simulink model "controller_tuner"  (R2016a)
settings: Solver=FixedStepDiscrete  StartTime=0.0  StopTime=inf  FixedStep=0.001  RelTol=1e-3
undefined symbols (not defined in the file or in its folder): Left_Leg
libraries: xpcethercatlib x14, slrtlib x5, simulink x2
settings Model: xpc_rtwmakecfg_data=_xpcethercatlib_  SimulationMode=external  Creator=Projectmarch  LastModifiedBy=Projectmarch
settings SolverCC: EnableConcurrentExecution=on
settings DataIOCC: SaveFormat=StructureWithTime
settings OptimizationCC: BlockReduction=off  OptimizeBlockIOStorage=off  BufferReuse=off  GlobalBufferReuse=off  ExpressionFolding=off  LocalBlockOutputs=off
settings HardwareCC: ProdBitPerPointer=32  ProdLargestAtomicFloat=None  ProdWordSize=32  ProdLongLongMode=on  ProdHWDeviceType=Generic->32-bit x86 compatible
settings RTWCC: SystemTargetFile=slrt.tlc  TemplateMakefile=slrt_default_tmf  Description=Simulink Real-Time  RTWCompilerOptimization=on

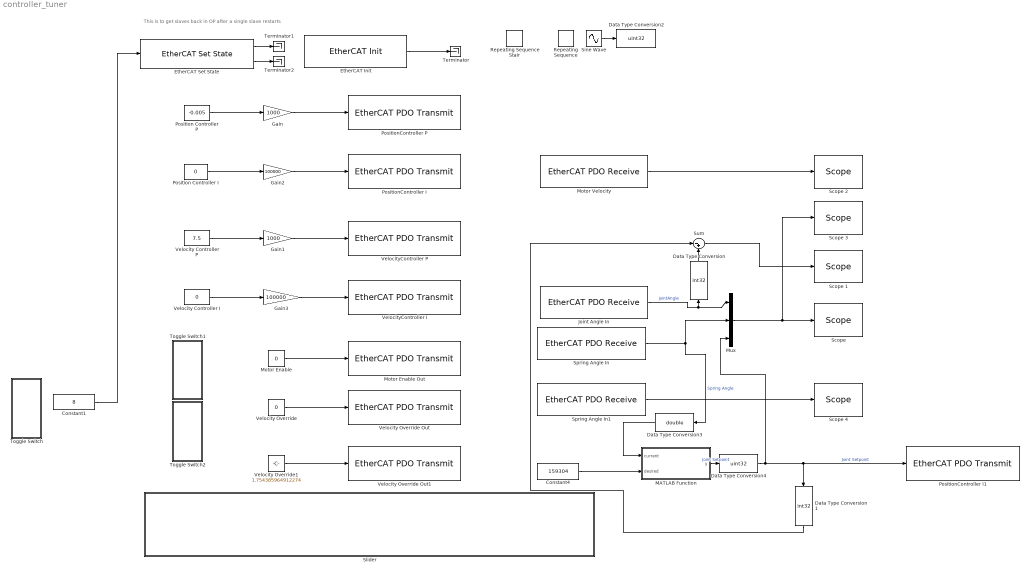
== system controller_tuner ==
  note: This is to get slaves back in OP after a single slave restarts
  Constant1 : Constant  Value=8  OutDataTypeStr=Inherit: Inherit via back propagation
  Constant4 : Constant  Value=159304  OutDataTypeStr=Inherit: Inherit via back propagation
  Data Type Conversion : DataTypeConversion  OutDataTypeStr=int32
  Data Type Conversion1 : DataTypeConversion  OutDataTypeStr=int32
  Data Type Conversion2 : DataTypeConversion  OutDataTypeStr=uint32
  Data Type Conversion3 : DataTypeConversion  OutDataTypeStr=double
  Data Type Conversion4 : DataTypeConversion  OutDataTypeStr=uint32
  "EtherCAT Init " : xpcethercatlib/EtherCAT Init   Priority=0  config_file=D:\Software\MATLAB\simulink-models\EtherCAT Config files\full_setup_v1.0.xml  device_id=0  pci_bus=2  pci_slot=0  dctuning=2  enaDebug=off  enaDC=on  errLink=off  masterDbg=off  stateChgDbg=off  baseClock=off  masterCfg=off  logFile='c:\dbglog.txt'  sample_time=0.001000
  "EtherCAT Set State " : xpcethercatlib/EtherCAT Set State   device_id=0  timeout=0  sample_time=0
  Gain : Gain  Gain=1000  OutDataTypeStr=Inherit: Inherit via back propagation
  Gain1 : Gain  Gain=1000  OutDataTypeStr=Inherit: Inherit via back propagation
  Gain2 : Gain  Gain=100000  OutDataTypeStr=Inherit: Inherit via back propagation
  Gain3 : Gain  Gain=100000  OutDataTypeStr=Inherit: Inherit via back propagation
  Joint Angle In : xpcethercatlib/EtherCAT PDO Receive  Priority=2  sig_name=Left_Leg.Inputs.H_jointAngle  sig_offset=1144  sig_type=uint32  type_size=32  sig_dim=1  device_id=0  sample_time=0.001000
  MATLAB Function : MATLAB Function  TreatAsAtomicUnit=on
  Motor Enable : Constant  Value=0  OutDataTypeStr=Inherit: Inherit via back propagation
  Motor Enable Out : xpcethercatlib/EtherCAT PDO Transmit   Priority=3  sig_name=Left_Leg.Outputs.H_motorEnable  sig_offset=1192  sig_type=uint8  type_size=8  sig_dim=1  device_id=0  sample_time=0.001000
  Motor Velocity : xpcethercatlib/EtherCAT PDO Receive  Priority=2  sig_name=Left_Leg.Inputs.H_motorVelocity  sig_offset=1224  sig_type=int16  type_size=16  sig_dim=1  device_id=0  sample_time=0.001000
  Mux : Mux  Inputs=3
  Position Controller I : Constant  Value=0
  Position Controller P : Constant  Value=-0.005
  PositionController I : xpcethercatlib/EtherCAT PDO Transmit   Priority=3  sig_name=Left_Leg.Outputs.H_data[1]  sig_offset=1304  sig_type=int32  type_size=32  sig_dim=1  device_id=0  sample_time=0.001000
  PositionController I1 : xpcethercatlib/EtherCAT PDO Transmit   Priority=3  sig_name=Left_Leg.Outputs.H_jointSetPoint  sig_offset=1160  sig_type=uint32  type_size=32  sig_dim=1  device_id=0  sample_time=0.001000
  PositionController P : xpcethercatlib/EtherCAT PDO Transmit   Priority=3  sig_name=Left_Leg.Outputs.H_data[0]  sig_offset=1272  sig_type=int32  type_size=32  sig_dim=1  device_id=0  sample_time=0.001000
  Repeating Sequence : simulink/Sources/Repeating Sequence  rep_seq_t=[0 2]  rep_seq_y=[0 2]
  Repeating Sequence Stair : simulink/Sources/Repeating Sequence Stair  OutValues=[3 1 4 2 1].'  tsamp=-1  OutMin=[]  OutMax=[]  OutDataTypeStr=double  OutputDataTypeScalingMode=double  OutDataType=fixdt(0,8)  ConRadixGroup=Best Precision: Vector-wise  OutScaling=2^-12
  "Scope " : slrtlib/Displays and Logging/Scope   scopeno=1  scopetype=Target  autostart=on  viewmode=Graphical sliding  formatstr='%15.6f'  grid=on  ylimits=[0,0]  nosamples=10000  noprepostsamples=0  interleave=1  triggermode=FreeRun  triggersignal=1  trigsignalfromport=off  triggerlevel=0.0  triggerslope=Either  triggerscope=1  triggersample=0  filename=data.dat  mode=Lazy  writesize=512  autorestart=off  dynamicfilemode=off  maxwritefilesize=512*1024^2
  Scope 1 : slrtlib/Displays and Logging/Scope   scopeno=2  scopetype=Target  autostart=on  viewmode=Graphical sliding  formatstr='%15.6f'  grid=on  ylimits=[0,0]  nosamples=10000  noprepostsamples=0  interleave=1  triggermode=FreeRun  triggersignal=1  trigsignalfromport=off  triggerlevel=0.0  triggerslope=Either  triggerscope=1  triggersample=0  filename=data.dat  mode=Lazy  writesize=512  autorestart=off  dynamicfilemode=off  maxwritefilesize=512*1024^2
  Scope 2 : slrtlib/Displays and Logging/Scope   scopeno=3  scopetype=Target  autostart=on  viewmode=Graphical sliding  formatstr='%15.6f'  grid=on  ylimits=[0,0]  nosamples=10000  noprepostsamples=0  interleave=1  triggermode=FreeRun  triggersignal=1  trigsignalfromport=off  triggerlevel=0.0  triggerslope=Either  triggerscope=1  triggersample=0  filename=data.dat  mode=Lazy  writesize=512  autorestart=off  dynamicfilemode=off  maxwritefilesize=512*1024^2
  Scope 3 : slrtlib/Displays and Logging/Scope   scopeno=4  scopetype=Target  autostart=on  viewmode=Numerical  formatstr='%15.6f'  grid=on  ylimits=[0,0]  nosamples=250  noprepostsamples=0  interleave=1  triggermode=FreeRun  triggersignal=1  trigsignalfromport=off  triggerlevel=0.0  triggerslope=Either  triggerscope=1  triggersample=0  filename=data.dat  mode=Lazy  writesize=512  autorestart=off  dynamicfilemode=off  maxwritefilesize=512*1024^2
  Scope 4 : slrtlib/Displays and Logging/Scope   scopeno=5  scopetype=Target  autostart=on  viewmode=Graphical sliding  formatstr='%15.6f'  grid=on  ylimits=[0,0]  nosamples=10000  noprepostsamples=0  interleave=1  triggermode=FreeRun  triggersignal=1  trigsignalfromport=off  triggerlevel=0.0  triggerslope=Either  triggerscope=1  triggersample=0  filename=data.dat  mode=Lazy  writesize=512  autorestart=off  dynamicfilemode=off  maxwritefilesize=512*1024^2
  Sine Wave : Sin  Amplitude=20000  Bias=370000  Frequency=2  SampleTime=0.001
  Slider : Subsystem  DialogController=hmiCreateDDGDialog  IsWebBlock=on  mask(MWDashboardBlock){webBlockId=69257127-0cdf-46c0-968c-0481a6079d56, webBlockType=slider, ShowInLibBrowser=on, ShowInitialText=on, HMISrcModelName=controller_tuner}
      mask prompts: webBlockId "WebBlock Id"; webBlockType "WebBlock Type"; HMISrcModelName "Source Model"
      mask Help: helpview([docroot '/mapfiles/simulink.map'], 'hmi_slider')
      mask Display:
      | if strcmp(get_param(bdroot(gcb),'BlockDiagramType'), 'library')
      |     image([(matlabroot) '/toolbox/simulink/hmi/icons/Slider.png']);
      | end
  Spring Angle In : xpcethercatlib/EtherCAT PDO Receive  Priority=2  sig_name=Left_Leg.Inputs.H_springAngle  sig_offset=1176  sig_type=uint32  type_size=32  sig_dim=1  device_id=0  sample_time=0.001000
  Spring Angle In1 : xpcethercatlib/EtherCAT PDO Receive  Priority=2  sig_name=Left_Leg.Inputs.K_footForceFront[0]  sig_offset=1464  sig_type=int32  type_size=32  sig_dim=1  device_id=0  sample_time=0.001000
  Sum : Sum  Inputs=|-+
  Terminator : Terminator
  Terminator1 : Terminator
  Terminator2 : Terminator
  Toggle Switch : Subsystem  DialogController=hmiCreateDDGDialog  IsWebBlock=on  mask(MWDashboardBlock){webBlockId=7114826d-f1c9-4545-bae4-963e2c516657, webBlockType=toggleswitch, ShowInLibBrowser=on, ShowInitialText=on, HMISrcModelName=controller_tuner}
      mask prompts: webBlockId "WebBlock Id"; webBlockType "WebBlock Type"; HMISrcModelName "Source Model"
      mask Help: helpview([docroot '/mapfiles/simulink.map'], 'hmi_toggle_switch')
      mask Display:
      | if strcmp(get_param(bdroot(gcb),'BlockDiagramType'), 'library')
      |     image([(matlabroot) '/toolbox/simulink/hmi/icons/ToggleSwitch.png']);
      | end
  Toggle Switch1 : Subsystem  DialogController=hmiCreateDDGDialog  IsWebBlock=on  mask(MWDashboardBlock){webBlockId=dae9756d-5b12-44cc-89b0-22c61f9c3f4a, webBlockType=toggleswitch, ShowInLibBrowser=on, ShowInitialText=on, HMISrcModelName=controller_tuner}
      mask prompts: webBlockId "WebBlock Id"; webBlockType "WebBlock Type"; HMISrcModelName "Source Model"
      mask Help: helpview([docroot '/mapfiles/simulink.map'], 'hmi_toggle_switch')
      mask Display:
      | if strcmp(get_param(bdroot(gcb),'BlockDiagramType'), 'library')
      |     image([(matlabroot) '/toolbox/simulink/hmi/icons/ToggleSwitch.png']);
      | end
  Toggle Switch2 : Subsystem  DialogController=hmiCreateDDGDialog  IsWebBlock=on  mask(MWDashboardBlock){webBlockId=6206497e-7561-4c19-9056-57079e110fb5, webBlockType=toggleswitch, ShowInLibBrowser=on, ShowInitialText=on, HMISrcModelName=controller_tuner}
      mask prompts: webBlockId "WebBlock Id"; webBlockType "WebBlock Type"; HMISrcModelName "Source Model"
      mask Help: helpview([docroot '/mapfiles/simulink.map'], 'hmi_toggle_switch')
      mask Display:
      | if strcmp(get_param(bdroot(gcb),'BlockDiagramType'), 'library')
      |     image([(matlabroot) '/toolbox/simulink/hmi/icons/ToggleSwitch.png']);
      | end
  Velocity Controller I : Constant  Value=0
  Velocity Controller P : Constant  Value=7.5
  Velocity Override : Constant  Value=0  OutDataTypeStr=Inherit: Inherit via back propagation
  Velocity Override Out : xpcethercatlib/EtherCAT PDO Transmit   Priority=3  sig_name=Left_Leg.Outputs.H_data[4]  sig_offset=1400  sig_type=int32  type_size=32  sig_dim=1  device_id=0  sample_time=0.001000
  Velocity Override Out1 : xpcethercatlib/EtherCAT PDO Transmit   Priority=3  sig_name=Left_Leg.Outputs.H_velocitySetPoint  sig_offset=1144  sig_type=int16  type_size=16  sig_dim=1  device_id=0  sample_time=0.001000
  Velocity Override1 : Constant  Value=1.754385964912274  OutDataTypeStr=Inherit: Inherit via back propagation
  VelocityController I : xpcethercatlib/EtherCAT PDO Transmit   Priority=3  sig_name=Left_Leg.Outputs.K_data[3]  sig_offset=1656  sig_type=int32  type_size=32  sig_dim=1  device_id=0  sample_time=0.001000
  VelocityController P : xpcethercatlib/EtherCAT PDO Transmit   Priority=3  sig_name=Left_Leg.Outputs.H_data[2]  sig_offset=1336  sig_type=int32  type_size=32  sig_dim=1  device_id=0  sample_time=0.001000
  wires:
  Position Controller P/1 -> Gain/1
  Gain/1 -> PositionController P/1
  Velocity Controller P/1 -> Gain1/1
  Gain1/1 -> VelocityController P/1
  Position Controller I/1 -> Gain2/1
  Velocity Controller I/1 -> Gain3/1
  Gain3/1 -> VelocityController I/1
  Gain2/1 -> PositionController I/1
  Velocity Override/1 -> Velocity Override Out/1
  Motor Enable/1 -> Motor Enable Out/1
  "EtherCAT Init "/1 -> Terminator/1
  Joint Angle In/1 -> Data Type Conversion/1, Mux/1  "jointAngle"
  Spring Angle In/1 -> Mux/2, Data Type Conversion3/1  "Spring Angle"
  Mux/1 -> Scope 3/1, "Scope "/1
  Motor Velocity/1 -> Scope 2/1
  Spring Angle In1/1 -> Scope 4/1
  Sum/1 -> Scope 1/1
  Data Type Conversion1/1 -> Sum/1
  Data Type Conversion/1 -> Sum/2
  Constant4/1 -> MATLAB Function/2(desired)
  Sine Wave/1 -> Data Type Conversion2/1
  "EtherCAT Set State "/1 -> Terminator1/1
  "EtherCAT Set State "/2 -> Terminator2/1
  Constant1/1 -> "EtherCAT Set State "/1
  Velocity Override1/1 -> Velocity Override Out1/1
  MATLAB Function/1(y) -> Data Type Conversion4/1  "Joint Setpoint"
  Data Type Conversion3/1 -> MATLAB Function/1(current)
  Data Type Conversion4/1 -> Mux/3, PositionController I1/1, Data Type Conversion1/1  "Joint Setpoint"

== system controller_tuner/Slider ==

== system controller_tuner/Toggle Switch ==

== system controller_tuner/Toggle Switch1 ==

== system controller_tuner/Toggle Switch2 ==

== matlab function controller_tuner/MATLAB Function ==
  data: current input; y output; desired input
function y = fcn(current,desired)
%#codegen

persistent i desiredPersistent trajectory startup;

f = 700;

if(isempty(trajectory))
   trajectory = [0 0]; 
end

% Send out the current value until desired is changed
if(isempty(startup))
    i = 1;
    startup = 1;
    desiredPersistent = desired;
end

% Same as above
if(desiredPersistent == desired && startup)
   y = current;
   return;
end

if(desiredPersistent ~= desired)
    i = 1;
    startup = 0;
    desiredPersistent = desired;
    trajectory = linspace(current,desiredPersistent,f);
end

if(i < length(trajectory))
    i = i+1;
end

y = trajectory(i);
